simulink model "Assignment_2_gamma_0point01"  (R2023b)
settings: Solver=ode45  StartTime=0.0  StopTime=100  MaxStep=2.0  RelTol=1e-3
libraries: dspfdesign x4
settings Model: Creator=User  LastModifiedBy=User

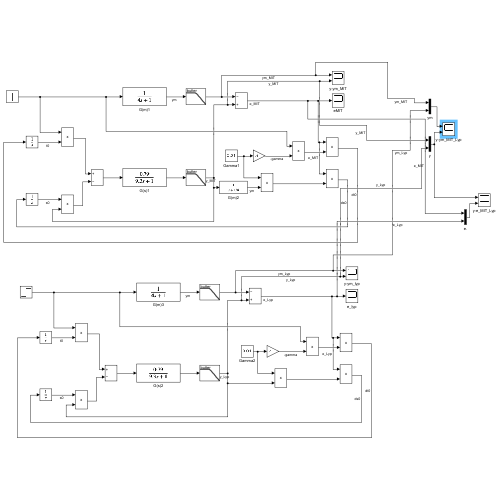
[thumbnail: Simulink's stored preview of the top-level diagram]
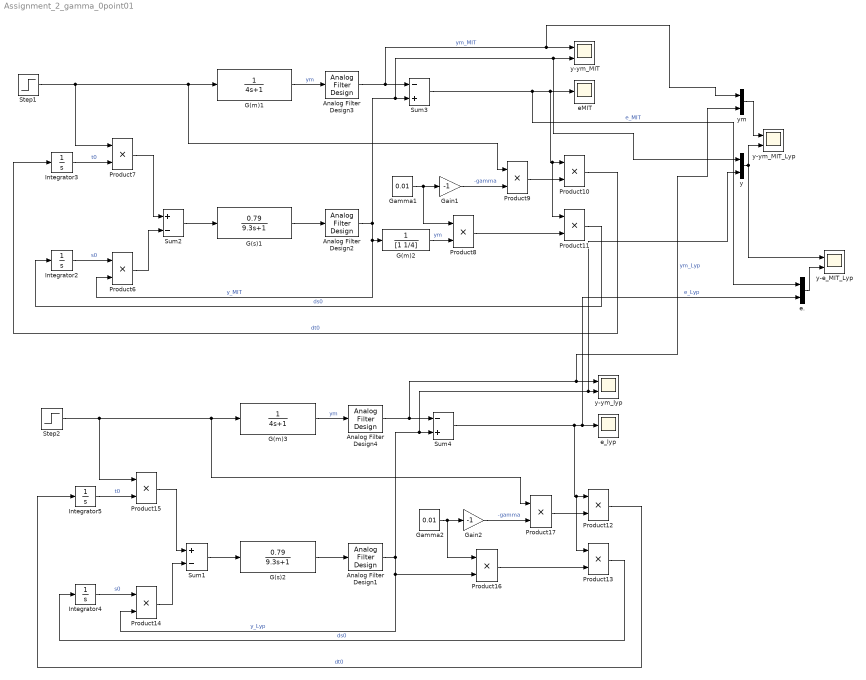
== system Assignment_2_gamma_0point01 ==
  Analog Filter Design{1..4} (4 alike) : dspfdesign/Analog Filter Design  method=Butterworth  filttype=Lowpass  N=4  Wlo=30  Whi=80  Rp=2  Rs=40
  G(m)1 : TransferFcn  Denominator=[4 1]
  G(m)2 : TransferFcn  Denominator=[1 1/4]
  G(m)3 : TransferFcn  Denominator=[4 1]
  G(s)1 : TransferFcn  Numerator=[0.79]  Denominator=[9.3 1]
  G(s)2 : TransferFcn  Numerator=[0.79]  Denominator=[9.3 1]
  Gain1 : Gain  Gain=-1
  Gain2 : Gain  Gain=-1
  Gamma1 : Constant  Value=0.01
  Gamma2 : Constant  Value=0.01
  Integrator{2..5} (4 alike) : Integrator
  Product{6..17} (12 alike) : Product
  Step1 : Step  Time=0  SampleTime=0
  Step2 : Step  Time=0  SampleTime=0
  Sum1 : Sum  Inputs=+-
  Sum2 : Sum  Inputs=+-
  Sum3 : Sum  Inputs=-+
  Sum4 : Sum  Inputs=-+
  e. : Mux  Inputs=2
  eMIT : Scope
  e_lyp : Scope
  y : Mux  Inputs=2
  y-e_MIT_Lyp : Scope  NumInputPorts=2
  y-ym_MIT : Scope  NumInputPorts=2
  y-ym_MIT_Lyp : Scope  NumInputPorts=2
  y-ym_lyp : Scope  NumInputPorts=2
  ym : Mux  Inputs=2
  wires:
  Integrator2/1 -> Product6/1  "s0"
  Product8/1 -> Product11/2
  Product7/1 -> Sum2/1
  Product9/1 -> Product10/2
  Sum3/1 -> e./1, Product11/1, Product10/1, eMIT/1  "e_MIT"
  Product11/1 -> Integrator2/1  "ds0"
  Integrator3/1 -> Product7/2  "t0"
  Gain1/1 -> Product9/2  "-gamma"
  Product10/1 -> Integrator3/1  "dt0"
  Gamma1/1 -> Product8/1, Gain1/1
  G(m)1/1 -> Analog Filter Design3/1  "ym"
  Step1/1 -> Product9/1, G(m)1/1, Product7/1
  G(s)1/1 -> Analog Filter Design2/1
  Analog Filter Design3/1 -> ym/1, y-ym_MIT/1, Sum3/1  "ym_MIT"
  Analog Filter Design2/1 -> G(m)2/1, Product6/2, y/1, y-ym_MIT/2, Sum3/2  "y_MIT"
  Product6/1 -> Sum2/2
  Sum2/1 -> G(s)1/1
  G(m)2/1 -> Product8/2  "ym"
  Integrator4/1 -> Product14/1  "s0"
  Product14/1 -> Sum1/2
  Product15/1 -> Sum1/1
  Integrator5/1 -> Product15/2  "t0"
  Sum4/1 -> Product13/1, Product12/1, e./2, e_lyp/1  "e_Lyp"
  Analog Filter Design1/1 -> Product14/2, Product16/2, y/2, y-ym_lyp/2, Sum4/2  "y_Lyp"
  Sum1/1 -> G(s)2/1
  G(s)2/1 -> Analog Filter Design1/1
  Gain2/1 -> Product17/2  "-gamma"
  Product12/1 -> Integrator5/1  "dt0"
  Product13/1 -> Integrator4/1  "ds0"
  G(m)3/1 -> Analog Filter Design4/1  "ym"
  Product17/1 -> Product12/2
  Step2/1 -> Product17/1, G(m)3/1, Product15/1
  Analog Filter Design4/1 -> ym/2, y-ym_lyp/1, Sum4/1  "ym_Lyp"
  Gamma2/1 -> Product16/1, Gain2/1
  Product16/1 -> Product13/2
  ym/1 -> y-ym_MIT_Lyp/1
  y/1 -> y-ym_MIT_Lyp/2, y-e_MIT_Lyp/1
  e./1 -> y-e_MIT_Lyp/2
